simulink model "Ideal_Comparison"  (R2023b)
settings: Solver=VariableStepAuto  StartTime=0.0  StopTime=11  RelTol=1e-3
InitFcn:
  | Ld = 0.000635;
  | Lq = 0.000635;
  | Rs = 0.05;
  | Lambda_m = 0.192;
  | J = 0.011;
  | P = 4;
  | B = 0.001889;
  | Kp = 0.5;
  | Ki = 55;
libraries: slpidlib x6, spsabctodq0Lib x2, SignalEditorBlockLib x1, spspowerguiLib x1
(part 1 of 2)
settings Model: Creator=Nabil  LastModifiedBy=Nabil

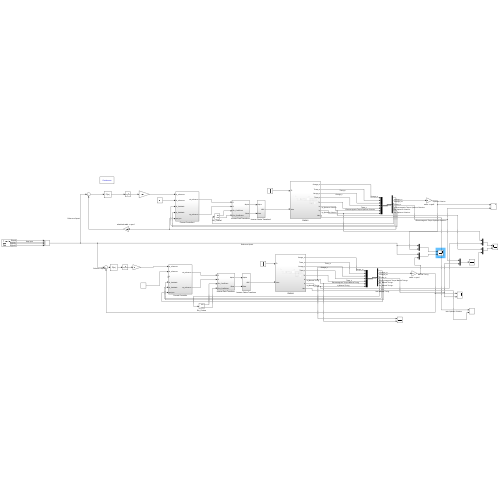
[thumbnail: Simulink's stored preview of the top-level diagram]
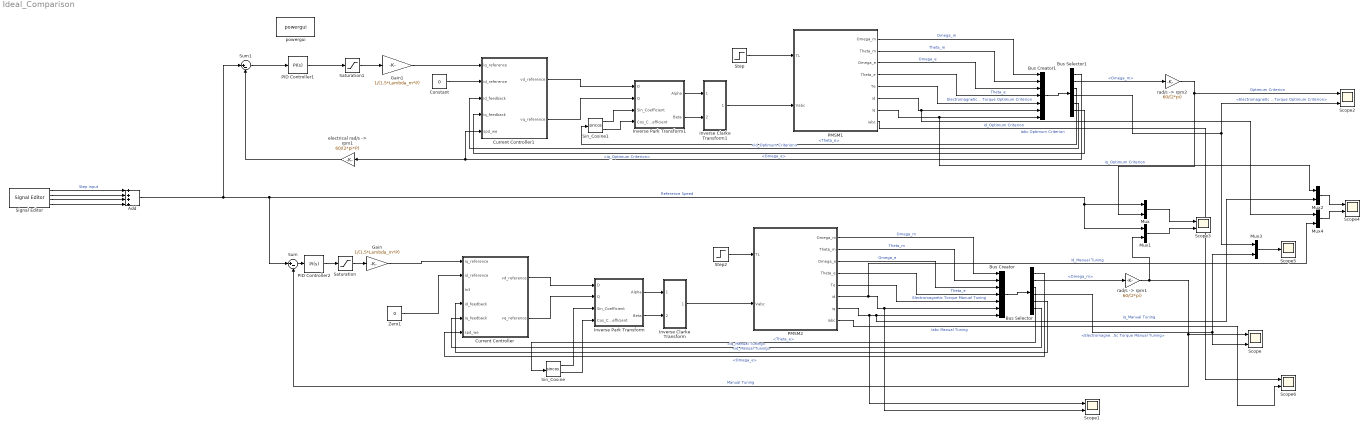
== system Ideal_Comparison ==
  Add : Sum  Inputs=++++
  Bus Creator : BusCreator  Inputs=7
  Bus Creator1 : BusCreator  Inputs=7
  Bus Selector : BusSelector  OutputSignals=Omega_e,Omega_m,Theta_e,Electromagnetic Torque Manual Tuning,id_Manual Tuning,iq_Manual Tuning
  Bus Selector1 : BusSelector  OutputSignals=Omega_e,Omega_m,Theta_e,Electromagnetic Torque Optimum Criterion,id_Optimum Criterion,iq_Optimum Criterion
  Constant : Constant  Value=0
  Current Controller : Subsystem
  Current Controller1 : Subsystem
  Gain : Gain  Gain=1/(1.5*Lambda_m*P)
  Gain1 : Gain  Gain=1/(1.5*Lambda_m*P)
  Inverse Clarke Transform : Subsystem
  Inverse Clarke Transform1 : Subsystem
  Inverse Park Transform : Subsystem
  Inverse Park Transform1 : Subsystem
  Mux{,1..4} (5 alike) : Mux  Inputs=2
  PID Controller1 : slpidlib/PID Controller  Controller=PI  Form=Parallel  TimeDomain=Continuous-time  UseExternalTs=off  SampleTime=-1  IntegratorMethod=Forward Euler  FilterMethod=Forward Euler  ControllerParametersSource=internal  P=0.218  I=2.25  UseKiTs=off  D=0  N=100  UseFilter=on  TunerSelectOption=Transfer Function Based (PID Tuner App)  InitialConditionSource=internal  InitialConditionForIntegrator=0  InitialConditionForFilter=0  DifferentiatorICPrevScaledInput=0  ExternalReset=none  TrackingMode=off  Kt=1  LimitOutput=off  SatLimitsSource=internal  UpperSaturationLimit=inf  LowerSaturationLimit=-inf  LinearizeAsGain=on  AntiWindupMode=none  Kb=1  LimitIntegrator=off  UpperIntegratorSaturationLimit=inf  LowerIntegratorSaturationLimit=-inf  POutMin=[]  POutMax=[]  IOutMin=[]  IOutMax=[]  DOutMin=[]  DOutMax=[]  NOutMin=[]  NOutMax=[]  SumOutMin=[]  SumOutMax=[]  SaturationOutMin=[]  SaturationOutMax=[]  PParamMin=[]  PParamMax=[]  IParamMin=[]  IParamMax=[]  DParamMin=[]  DParamMax=[]  NParamMin=[]  NParamMax=[]  KbParamMin=[]  KbParamMax=[]  KtParamMin=[]  KtParamMax=[]  KbOutMin=[]  KbOutMax=[]  KtOutMin=[]  KtOutMax=[]  IntegratorOutMin=[]  IntegratorOutMax=[]  FilterOutMin=[]  FilterOutMax=[]  SumI1OutMin=[]  SumI1OutMax=[]  SumI2OutMin=[]  SumI2OutMax=[]  SumI3OutMin=[]  SumI3OutMax=[]  SumI4OutMin=[]  SumI4OutMax=[]  SumDOutMin=[]  SumDOutMax=[]  DifferentiatorOutMin=[]  DifferentiatorOutMax=[]  FilterDiffOutCoefMin=[]  FilterDiffOutCoefMax=[]  ReciprocalOutMin=[]  ReciprocalOutMax=[]  SumDenOutMin=[]  SumDenOutMax=[]  SumNumOutMin=[]  SumNumOutMax=[]  DivideOutMin=[]  DivideOutMax=[]  UdiffTsProdOutMin=[]  UdiffTsProdOutMax=[]  NTsProdOutMin=[]  NTsProdOutMax=[]  UintegralTsProdOutMin=[]  UintegralTsProdOutMax=[]  UngainTsProdOutMin=[]  UngainTsProdOutMax=[]  ClampingZeroOutDataTypeStr=Inherit: Inherit via back propagation  ClampingZeroOutMin=[]  ClampingZeroOutMax=[]  FilterDenConstantOutDataTypeStr=Inherit: Inherit via back propagation  FilterDenConstantOutMin=[]  FilterDenConstantOutMax=[]  PCopyOutDataTypeStr=Inherit: Inherit via back propagation  PCopyOutMin=[]  PCopyOutMax=[]  NCopyOutDataTypeStr=Inherit: Inherit via back propagation  NCopyOutMin=[]  NCopyOutMax=[]  IntegratorContinuousStateAttributes=''  IntegratorStateMustResolveToSignalObject=off  IntegratorRTWStateStorageClass=Auto  FilterContinuousStateAttributes=''  FilterStateMustResolveToSignalObject=off  FilterRTWStateStorageClass=Auto  ParallelPVariant=InternalParameters  IdealPVariant=Disabled  IVariant=InternalParameters  DVariant=Disabled  IntegratorVariant=Continuous  SatVariant=Disabled  AWVariant=Passthrough  PCopyVariant=Disabled  TRVariant=Disabled  FdbkBlocksVariant=Forward  IdealPFdbkVariant=Disabled  SatFdbkVariant=Disabled  DerivativeFilterVariant=Disabled  NVariant=Disabled  NCopyVariant=Disabled_SignalSpec  FilterICVariant=Disabled  IntegratorICVariant=InternalICs  ExternalResetVariant=Disabled  TRSumVariant=Passthrough  SumFdbkVariant=Disabled  SumVariant=Sum_PI  TsampFilterVariant=InternalTs  TsampNgainVariant=Passthrough  TsampIntegralVariant=Disabled_SignalSpec  ExternalSaturationOutDataTypeStr=Inherit: Same as second input
  PID Controller2 : slpidlib/PID Controller  Controller=PI  Form=Parallel  TimeDomain=Continuous-time  UseExternalTs=off  SampleTime=-1  IntegratorMethod=Forward Euler  FilterMethod=Forward Euler  ControllerParametersSource=internal  P=0.3283  I=2.54  UseKiTs=off  D=0  N=100  UseFilter=on  TunerSelectOption=Transfer Function Based (PID Tuner App)  InitialConditionSource=internal  InitialConditionForIntegrator=0  InitialConditionForFilter=0  DifferentiatorICPrevScaledInput=0  ExternalReset=none  TrackingMode=off  Kt=1  LimitOutput=off  SatLimitsSource=internal  UpperSaturationLimit=inf  LowerSaturationLimit=-inf  LinearizeAsGain=on  AntiWindupMode=none  Kb=1  LimitIntegrator=off  UpperIntegratorSaturationLimit=inf  LowerIntegratorSaturationLimit=-inf  POutMin=[]  POutMax=[]  IOutMin=[]  IOutMax=[]  DOutMin=[]  DOutMax=[]  NOutMin=[]  NOutMax=[]  SumOutMin=[]  SumOutMax=[]  SaturationOutMin=[]  SaturationOutMax=[]  PParamMin=[]  PParamMax=[]  IParamMin=[]  IParamMax=[]  DParamMin=[]  DParamMax=[]  NParamMin=[]  NParamMax=[]  KbParamMin=[]  KbParamMax=[]  KtParamMin=[]  KtParamMax=[]  KbOutMin=[]  KbOutMax=[]  KtOutMin=[]  KtOutMax=[]  IntegratorOutMin=[]  IntegratorOutMax=[]  FilterOutMin=[]  FilterOutMax=[]  SumI1OutMin=[]  SumI1OutMax=[]  SumI2OutMin=[]  SumI2OutMax=[]  SumI3OutMin=[]  SumI3OutMax=[]  SumI4OutMin=[]  SumI4OutMax=[]  SumDOutMin=[]  SumDOutMax=[]  DifferentiatorOutMin=[]  DifferentiatorOutMax=[]  FilterDiffOutCoefMin=[]  FilterDiffOutCoefMax=[]  ReciprocalOutMin=[]  ReciprocalOutMax=[]  SumDenOutMin=[]  SumDenOutMax=[]  SumNumOutMin=[]  SumNumOutMax=[]  DivideOutMin=[]  DivideOutMax=[]  UdiffTsProdOutMin=[]  UdiffTsProdOutMax=[]  NTsProdOutMin=[]  NTsProdOutMax=[]  UintegralTsProdOutMin=[]  UintegralTsProdOutMax=[]  UngainTsProdOutMin=[]  UngainTsProdOutMax=[]  ClampingZeroOutDataTypeStr=Inherit: Inherit via back propagation  ClampingZeroOutMin=[]  ClampingZeroOutMax=[]  FilterDenConstantOutDataTypeStr=Inherit: Inherit via back propagation  FilterDenConstantOutMin=[]  FilterDenConstantOutMax=[]  PCopyOutDataTypeStr=Inherit: Inherit via back propagation  PCopyOutMin=[]  PCopyOutMax=[]  NCopyOutDataTypeStr=Inherit: Inherit via back propagation  NCopyOutMin=[]  NCopyOutMax=[]  IntegratorContinuousStateAttributes=''  IntegratorStateMustResolveToSignalObject=off  IntegratorRTWStateStorageClass=Auto  FilterContinuousStateAttributes=''  FilterStateMustResolveToSignalObject=off  FilterRTWStateStorageClass=Auto  ParallelPVariant=InternalParameters  IdealPVariant=Disabled  IVariant=InternalParameters  DVariant=Disabled  IntegratorVariant=Continuous  SatVariant=Disabled  AWVariant=Passthrough  PCopyVariant=Disabled  TRVariant=Disabled  FdbkBlocksVariant=Forward  IdealPFdbkVariant=Disabled  SatFdbkVariant=Disabled  DerivativeFilterVariant=Disabled  NVariant=Disabled  NCopyVariant=Disabled_SignalSpec  FilterICVariant=Disabled  IntegratorICVariant=InternalICs  ExternalResetVariant=Disabled  TRSumVariant=Passthrough  SumFdbkVariant=Disabled  SumVariant=Sum_PI  TsampFilterVariant=InternalTs  TsampNgainVariant=Passthrough  TsampIntegralVariant=Disabled_SignalSpec  ExternalSaturationOutDataTypeStr=Inherit: Same as second input
  PMSM1 : Subsystem
  PMSM2 : Subsystem
  Saturation : Saturate  UpperLimit=111  LowerLimit=-126
  Saturation1 : Saturate  UpperLimit=111  LowerLimit=-126
  Scope{,1..4,6} (6 alike) : Scope  NumInputPorts=2
  Scope5 : Scope
  Signal Editor : SignalEditorBlockLib/Signal Editor  FileName=D:\Semester 8\Files\Modeling 24_2_2024\Signal3.mat  ActiveScenario=Scenario  ActiveSignal=Signal  IsBus=off  OutputBusObjectStr=Bus: BusObject  SampleTime=0  Interpolate=off  ZeroCross=off  OutputAfterFinalValue=Setting to zero  Unit=inherit  PreserveSignalName=on  ApplySigPropsToAllScenarios=on  ApplySigPropsToAllSignals=off
  Sin_Cosine : Trigonometry  Operator=sincos
  Sin_Cosine1 : Trigonometry  Operator=sincos
  Step : Step  Before=10  After=35  SampleTime=0
  Step2 : Step  Before=10  After=35  SampleTime=0
  Sum : Sum  Inputs=|+-
  Sum1 : Sum  Inputs=|+-
  Zero1 : Constant  Value=0  OutDataTypeStr=Inherit: Inherit via back propagation
  "electrical rad/s -> rpm1" : Gain  Gain=60/(2*pi*P)
  powergui : spspowerguiLib/powergui  Priority=1  SimulationMode=Continuous  SampleTime=50e-6  frequency=60  Iterations=50  frequencyindice=0  Pbase=100e6  ErrMax=1e-4  UnitsV=kV  UnitsW=MW  buscounter=0  FunctionMessages=off  echomessages=off  EnableUseOfTLC=off  CurrentSourceSwitches=off  DisableSnubberDevices=off  DisableRonSwitches=off  DisableVfSwitches=off  DisplayEquations=off  AutomaticDiscreteSolvers=off  SolverType=Tustin/Backward Euler (TBE)  Interpol=off  ExternalGateDelay=off  methode=off  Ts=100  x0status=blocks  SPID=on  SwTol=0  HookPort=off  NonlinearTolerance=1e-4  nMaxIteration=100  ContinueOnMaxIteration=off  RestoreLinks=warning  ResistiveCurrentMeasurement=off  Frange=[0:2:500]  Ylog=off  Xlog=on  ShowGrid=off  save=off  variable=ZData  structure=0  ZoomFFT=off  StartTime=0.0  cycles=1  DisplayStyle=1  fundamental=60  FreqAxis=off  MaxFrequency=1000  frequencyindicesteady=1  RmsSteady=1  display=off
  "rad/s -> rpm1" : Gain  Gain=60/(2*pi)
  "rad/s -> rpm2" : Gain  Gain=60/(2*pi)
  wires:
  PMSM2/2(Theta_m) -> Bus Creator/2  "Theta_m"
  Bus Selector/4 -> Mux3/2, Scope/2  "<Electromagnetic Torque Manual Tuning>"
  Bus Selector/1 -> Current Controller/6(spd_we)  "<Omega_e>"
  PMSM2/3(Omega_e) -> Bus Creator/3  "Omega_e"
  PMSM2/6(id) -> Mux4/2, Scope1/2, Bus Creator/6  "id_Manual Tuning"
  PMSM2/7(iq) -> Scope1/1, Mux2/2, Bus Creator/7  "iq_Manual Tuning"
  PMSM2/5(Te) -> Bus Creator/5  "Electromagnetic Torque Manual Tuning"
  Gain/1 -> Current Controller/1(iq_reference)
  Sin_Cosine/1 -> Inverse Park Transform/3(Sin_Coefficient)
  Bus Selector/3 -> Sin_Cosine/1  "<Theta_e>"
  Inverse Park Transform/1(Alpha) -> Inverse Clarke Transform/1(Alpha)
  Current Controller/2(vq_reference) -> Inverse Park Transform/2(Q)
  Bus Selector/6 -> Current Controller/5(iq_feedback)  "<iq_Manual Tuning>"
  Bus Creator/1 -> Bus Selector/1
  Step2/1 -> PMSM2/1(TL)
  "rad/s -> rpm1"/1 -> Mux1/2, Scope/1, Sum/2  "Manual Tuning"
  Inverse Clarke Transform/1(ABC) -> PMSM2/2(Vabc)
  Sin_Cosine/2 -> Inverse Park Transform/4(Cos_Coefficient)
  Inverse Park Transform/2(Beta) -> Inverse Clarke Transform/2(Beta)
  Bus Selector/5 -> Current Controller/4(id_feedback)  "<id_Manual Tuning>"
  Bus Selector/2 -> "rad/s -> rpm1"/1  "<Omega_m>"
  PMSM2/4(Theta_e) -> Bus Creator/4  "Theta_e"
  Zero1/1 -> Current Controller/2(id_reference)
  Current Controller/1(vd_reference) -> Inverse Park Transform/1(D)
  PMSM2/1(Omega_m) -> Bus Creator/1  "Omega_m"
  PID Controller2/1 -> Saturation/1
  Sum/1 -> PID Controller2/1
  Saturation/1 -> Gain/1
  Signal Editor/1 -> Add/1  "Step input"
  PMSM1/2(Theta_m) -> Bus Creator1/2  "Theta_m"
  Bus Selector1/4 -> Mux3/1, Scope2/2  "<Electromagnetic Torque Optimum Criterion>"
  Bus Selector1/1 -> Current Controller1/5(spd_we), "electrical rad/s -> rpm1"/1  "<Omega_e>"
  PMSM1/3(Omega_e) -> Bus Creator1/3  "Omega_e"
  "electrical rad/s -> rpm1"/1 -> Sum1/2
  PMSM1/6(id) -> Mux4/1, Bus Creator1/6  "id_Optimum Criterion"
  Saturation1/1 -> Gain1/1
  Sin_Cosine1/1 -> Inverse Park Transform1/3(Sin_Coefficient)
  PMSM1/7(iq) -> Mux2/1, Bus Creator1/7  "iq_Optimum Criterion"
  PMSM1/5(Te) -> Bus Creator1/5  "Electromagnetic Torque Optimum Criterion"
  Bus Selector1/3 -> Sin_Cosine1/1  "<Theta_e>"
  Inverse Park Transform1/1(Alpha) -> Inverse Clarke Transform1/1(Alpha)
  Current Controller1/2(vq_reference) -> Inverse Park Transform1/2(Q)
  Gain1/1 -> Current Controller1/1(iq_reference)
  Bus Selector1/6 -> Current Controller1/4(iq_feedback)  "<iq_Optimum Criterion>"
  Bus Creator1/1 -> Bus Selector1/1
  Step/1 -> PMSM1/1(TL)
  "rad/s -> rpm2"/1 -> Mux/2, Scope2/1  "Optimum Criterion"
  Inverse Clarke Transform1/1(ABC) -> PMSM1/2(Vabc)
  Sin_Cosine1/2 -> Inverse Park Transform1/4(Cos_Coefficient)
  Inverse Park Transform1/2(Beta) -> Inverse Clarke Transform1/2(Beta)
  Bus Selector1/5 -> Current Controller1/3(id_feedback)  "<id_Optimum Criterion>"
  Bus Selector1/2 -> "rad/s -> rpm2"/1  "<Omega_m>"
  PMSM1/4(Theta_e) -> Bus Creator1/4  "Theta_e"
  Constant/1 -> Current Controller1/2(id_reference)
  Current Controller1/1(vd_reference) -> Inverse Park Transform1/1(D)
  PMSM1/1(Omega_m) -> Bus Creator1/1  "Omega_m"
  Mux/1 -> Scope3/1
  Mux1/1 -> Scope3/2
  Mux3/1 -> Scope5/1
  Mux4/1 -> Scope4/2
  Mux2/1 -> Scope4/1
  PMSM1/8(iabc) -> Scope6/1  "Iabc Optimum Criterion"
  PMSM2/8(iabc) -> Scope6/2  "Iabc Manual Tuning"
  Sum1/1 -> PID Controller1/1
  PID Controller1/1 -> Saturation1/1
  Signal Editor/2 -> Add/2
  Add/1 -> Sum1/1, Sum/1, Mux1/1, Mux/1  "Reference Speed"
  Signal Editor/3 -> Add/3
  Signal Editor/4 -> Add/4

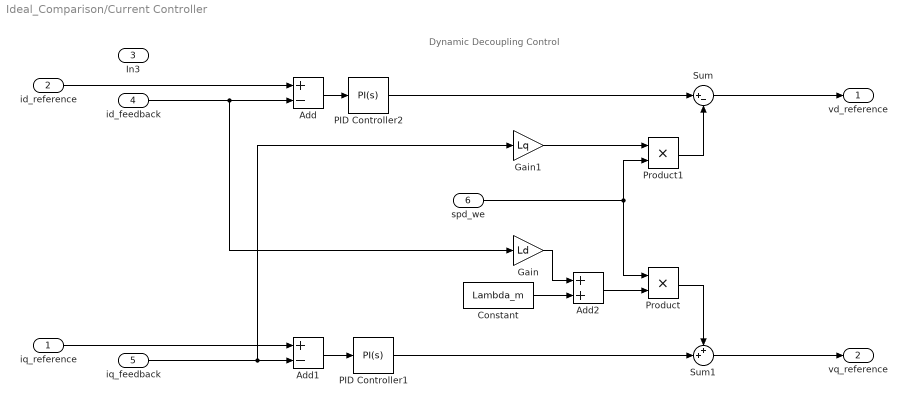
== system Ideal_Comparison/Current Controller ==
  note: Dynamic Decoupling Control
  iq_reference : Inport  SampleTime=1e-4
  id_reference : Inport  Port=2  SampleTime=1e-4
  In3 : Inport  Port=3
  id_feedback : Inport  Port=4  SampleTime=1e-4
  iq_feedback : Inport  Port=5  SampleTime=1e-4
  spd_we : Inport  Port=6  SampleTime=1e-4
  Add : Sum  Inputs=+-
  Add1 : Sum  Inputs=+-
  Add2 : Sum
  Constant : Constant  Value=Lambda_m  SampleTime=1e-4
  Gain : Gain  Gain=Ld
  Gain1 : Gain  Gain=Lq
  PID Controller1 : slpidlib/PID Controller  Controller=PI  Form=Parallel  TimeDomain=Continuous-time  UseExternalTs=off  SampleTime=-1  IntegratorMethod=Forward Euler  FilterMethod=Forward Euler  ControllerParametersSource=internal  P=0.5  I=53  UseKiTs=off  D=0  N=100  UseFilter=on  TunerSelectOption=Transfer Function Based (PID Tuner App)  InitialConditionSource=internal  InitialConditionForIntegrator=0  InitialConditionForFilter=0  DifferentiatorICPrevScaledInput=0  ExternalReset=none  TrackingMode=off  Kt=1  LimitOutput=off  SatLimitsSource=internal  UpperSaturationLimit=inf  LowerSaturationLimit=-inf  LinearizeAsGain=on  AntiWindupMode=none  Kb=1  LimitIntegrator=off  UpperIntegratorSaturationLimit=inf  LowerIntegratorSaturationLimit=-inf  POutMin=[]  POutMax=[]  IOutMin=[]  IOutMax=[]  DOutMin=[]  DOutMax=[]  NOutMin=[]  NOutMax=[]  SumOutMin=[]  SumOutMax=[]  SaturationOutMin=[]  SaturationOutMax=[]  PParamMin=[]  PParamMax=[]  IParamMin=[]  IParamMax=[]  DParamMin=[]  DParamMax=[]  NParamMin=[]  NParamMax=[]  KbParamMin=[]  KbParamMax=[]  KtParamMin=[]  KtParamMax=[]  KbOutMin=[]  KbOutMax=[]  KtOutMin=[]  KtOutMax=[]  IntegratorOutMin=[]  IntegratorOutMax=[]  FilterOutMin=[]  FilterOutMax=[]  SumI1OutMin=[]  SumI1OutMax=[]  SumI2OutMin=[]  SumI2OutMax=[]  SumI3OutMin=[]  SumI3OutMax=[]  SumI4OutMin=[]  SumI4OutMax=[]  SumDOutMin=[]  SumDOutMax=[]  DifferentiatorOutMin=[]  DifferentiatorOutMax=[]  FilterDiffOutCoefMin=[]  FilterDiffOutCoefMax=[]  ReciprocalOutMin=[]  ReciprocalOutMax=[]  SumDenOutMin=[]  SumDenOutMax=[]  SumNumOutMin=[]  SumNumOutMax=[]  DivideOutMin=[]  DivideOutMax=[]  UdiffTsProdOutMin=[]  UdiffTsProdOutMax=[]  NTsProdOutMin=[]  NTsProdOutMax=[]  UintegralTsProdOutMin=[]  UintegralTsProdOutMax=[]  UngainTsProdOutMin=[]  UngainTsProdOutMax=[]  ClampingZeroOutDataTypeStr=Inherit: Inherit via back propagation  ClampingZeroOutMin=[]  ClampingZeroOutMax=[]  FilterDenConstantOutDataTypeStr=Inherit: Inherit via back propagation  FilterDenConstantOutMin=[]  FilterDenConstantOutMax=[]  PCopyOutDataTypeStr=Inherit: Inherit via back propagation  PCopyOutMin=[]  PCopyOutMax=[]  NCopyOutDataTypeStr=Inherit: Inherit via back propagation  NCopyOutMin=[]  NCopyOutMax=[]  IntegratorContinuousStateAttributes=''  IntegratorStateMustResolveToSignalObject=off  IntegratorRTWStateStorageClass=Auto  FilterContinuousStateAttributes=''  FilterStateMustResolveToSignalObject=off  FilterRTWStateStorageClass=Auto  ParallelPVariant=InternalParameters  IdealPVariant=Disabled  IVariant=InternalParameters  DVariant=Disabled  IntegratorVariant=Continuous  SatVariant=Disabled  AWVariant=Passthrough  PCopyVariant=Disabled  TRVariant=Disabled  FdbkBlocksVariant=Forward  IdealPFdbkVariant=Disabled  SatFdbkVariant=Disabled  DerivativeFilterVariant=Disabled  NVariant=Disabled  NCopyVariant=Disabled_SignalSpec  FilterICVariant=Disabled  IntegratorICVariant=InternalICs  ExternalResetVariant=Disabled  TRSumVariant=Passthrough  SumFdbkVariant=Disabled  SumVariant=Sum_PI  TsampFilterVariant=InternalTs  TsampNgainVariant=Passthrough  TsampIntegralVariant=Disabled_SignalSpec  ExternalSaturationOutDataTypeStr=Inherit: Same as second input
  PID Controller2 : slpidlib/PID Controller  Controller=PI  Form=Parallel  TimeDomain=Continuous-time  UseExternalTs=off  SampleTime=-1  IntegratorMethod=Forward Euler  FilterMethod=Forward Euler  ControllerParametersSource=internal  P=0.5  I=53  UseKiTs=off  D=0  N=100  UseFilter=on  TunerSelectOption=Transfer Function Based (PID Tuner App)  InitialConditionSource=internal  InitialConditionForIntegrator=0  InitialConditionForFilter=0  DifferentiatorICPrevScaledInput=0  ExternalReset=none  TrackingMode=off  Kt=1  LimitOutput=off  SatLimitsSource=internal  UpperSaturationLimit=inf  LowerSaturationLimit=-inf  LinearizeAsGain=on  AntiWindupMode=none  Kb=1  LimitIntegrator=off  UpperIntegratorSaturationLimit=inf  LowerIntegratorSaturationLimit=-inf  POutMin=[]  POutMax=[]  IOutMin=[]  IOutMax=[]  DOutMin=[]  DOutMax=[]  NOutMin=[]  NOutMax=[]  SumOutMin=[]  SumOutMax=[]  SaturationOutMin=[]  SaturationOutMax=[]  PParamMin=[]  PParamMax=[]  IParamMin=[]  IParamMax=[]  DParamMin=[]  DParamMax=[]  NParamMin=[]  NParamMax=[]  KbParamMin=[]  KbParamMax=[]  KtParamMin=[]  KtParamMax=[]  KbOutMin=[]  KbOutMax=[]  KtOutMin=[]  KtOutMax=[]  IntegratorOutMin=[]  IntegratorOutMax=[]  FilterOutMin=[]  FilterOutMax=[]  SumI1OutMin=[]  SumI1OutMax=[]  SumI2OutMin=[]  SumI2OutMax=[]  SumI3OutMin=[]  SumI3OutMax=[]  SumI4OutMin=[]  SumI4OutMax=[]  SumDOutMin=[]  SumDOutMax=[]  DifferentiatorOutMin=[]  DifferentiatorOutMax=[]  FilterDiffOutCoefMin=[]  FilterDiffOutCoefMax=[]  ReciprocalOutMin=[]  ReciprocalOutMax=[]  SumDenOutMin=[]  SumDenOutMax=[]  SumNumOutMin=[]  SumNumOutMax=[]  DivideOutMin=[]  DivideOutMax=[]  UdiffTsProdOutMin=[]  UdiffTsProdOutMax=[]  NTsProdOutMin=[]  NTsProdOutMax=[]  UintegralTsProdOutMin=[]  UintegralTsProdOutMax=[]  UngainTsProdOutMin=[]  UngainTsProdOutMax=[]  ClampingZeroOutDataTypeStr=Inherit: Inherit via back propagation  ClampingZeroOutMin=[]  ClampingZeroOutMax=[]  FilterDenConstantOutDataTypeStr=Inherit: Inherit via back propagation  FilterDenConstantOutMin=[]  FilterDenConstantOutMax=[]  PCopyOutDataTypeStr=Inherit: Inherit via back propagation  PCopyOutMin=[]  PCopyOutMax=[]  NCopyOutDataTypeStr=Inherit: Inherit via back propagation  NCopyOutMin=[]  NCopyOutMax=[]  IntegratorContinuousStateAttributes=''  IntegratorStateMustResolveToSignalObject=off  IntegratorRTWStateStorageClass=Auto  FilterContinuousStateAttributes=''  FilterStateMustResolveToSignalObject=off  FilterRTWStateStorageClass=Auto  ParallelPVariant=InternalParameters  IdealPVariant=Disabled  IVariant=InternalParameters  DVariant=Disabled  IntegratorVariant=Continuous  SatVariant=Disabled  AWVariant=Passthrough  PCopyVariant=Disabled  TRVariant=Disabled  FdbkBlocksVariant=Forward  IdealPFdbkVariant=Disabled  SatFdbkVariant=Disabled  DerivativeFilterVariant=Disabled  NVariant=Disabled  NCopyVariant=Disabled_SignalSpec  FilterICVariant=Disabled  IntegratorICVariant=InternalICs  ExternalResetVariant=Disabled  TRSumVariant=Passthrough  SumFdbkVariant=Disabled  SumVariant=Sum_PI  TsampFilterVariant=InternalTs  TsampNgainVariant=Passthrough  TsampIntegralVariant=Disabled_SignalSpec  ExternalSaturationOutDataTypeStr=Inherit: Same as second input
  Product : Product
  Product1 : Product
  Sum : Sum  Inputs=|+-
  Sum1 : Sum  Inputs=++|
  vd_reference : Outport  SampleTime=1e-4  VectorParamsAs1DForOutWhenUnconnected=off
  vq_reference : Outport  Port=2  SampleTime=1e-4  VectorParamsAs1DForOutWhenUnconnected=off
  wires:
  Sum/1 -> vd_reference/1
  PID Controller2/1 -> Sum/1
  id_feedback/1 -> Gain/1, Add/2
  Add/1 -> PID Controller2/1
  iq_feedback/1 -> Gain1/1, Add1/2
  id_reference/1 -> Add/1
  Add1/1 -> PID Controller1/1
  iq_reference/1 -> Add1/1
  Sum1/1 -> vq_reference/1
  PID Controller1/1 -> Sum1/2
  Gain/1 -> Add2/1
  Constant/1 -> Add2/2
  Add2/1 -> Product/2
  spd_we/1 -> Product1/2, Product/1
  Gain1/1 -> Product1/1
  Product1/1 -> Sum/2
  Product/1 -> Sum1/1

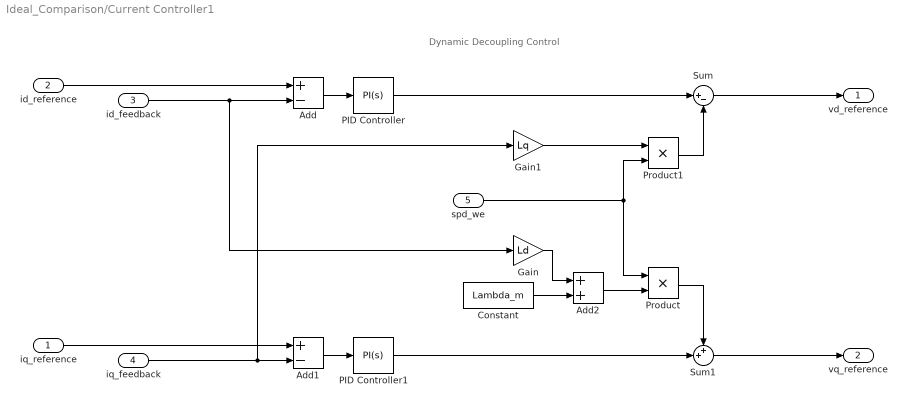
== system Ideal_Comparison/Current Controller1 ==
  note: Dynamic Decoupling Control
  iq_reference : Inport  SampleTime=1e-4
  id_reference : Inport  Port=2  SampleTime=1e-4
  id_feedback : Inport  Port=3  SampleTime=1e-4
  iq_feedback : Inport  Port=4  SampleTime=1e-4
  spd_we : Inport  Port=5  SampleTime=1e-4
  Add : Sum  Inputs=+-
  Add1 : Sum  Inputs=+-
  Add2 : Sum
  Constant : Constant  Value=Lambda_m  SampleTime=1e-4
  Gain : Gain  Gain=Ld
  Gain1 : Gain  Gain=Lq
  PID Controller : slpidlib/PID Controller  Controller=PI  Form=Parallel  TimeDomain=Continuous-time  UseExternalTs=off  SampleTime=-1  IntegratorMethod=Forward Euler  FilterMethod=Forward Euler  ControllerParametersSource=internal  P=7.9735  I=625  UseKiTs=off  D=0  N=100  UseFilter=on  TunerSelectOption=Transfer Function Based (PID Tuner App)  InitialConditionSource=internal  InitialConditionForIntegrator=0  InitialConditionForFilter=0  DifferentiatorICPrevScaledInput=0  ExternalReset=none  TrackingMode=off  Kt=1  LimitOutput=off  SatLimitsSource=internal  UpperSaturationLimit=inf  LowerSaturationLimit=-inf  LinearizeAsGain=on  AntiWindupMode=none  Kb=1  LimitIntegrator=off  UpperIntegratorSaturationLimit=inf  LowerIntegratorSaturationLimit=-inf  POutMin=[]  POutMax=[]  IOutMin=[]  IOutMax=[]  DOutMin=[]  DOutMax=[]  NOutMin=[]  NOutMax=[]  SumOutMin=[]  SumOutMax=[]  SaturationOutMin=[]  SaturationOutMax=[]  PParamMin=[]  PParamMax=[]  IParamMin=[]  IParamMax=[]  DParamMin=[]  DParamMax=[]  NParamMin=[]  NParamMax=[]  KbParamMin=[]  KbParamMax=[]  KtParamMin=[]  KtParamMax=[]  KbOutMin=[]  KbOutMax=[]  KtOutMin=[]  KtOutMax=[]  IntegratorOutMin=[]  IntegratorOutMax=[]  FilterOutMin=[]  FilterOutMax=[]  SumI1OutMin=[]  SumI1OutMax=[]  SumI2OutMin=[]  SumI2OutMax=[]  SumI3OutMin=[]  SumI3OutMax=[]  SumI4OutMin=[]  SumI4OutMax=[]  SumDOutMin=[]  SumDOutMax=[]  DifferentiatorOutMin=[]  DifferentiatorOutMax=[]  FilterDiffOutCoefMin=[]  FilterDiffOutCoefMax=[]  ReciprocalOutMin=[]  ReciprocalOutMax=[]  SumDenOutMin=[]  SumDenOutMax=[]  SumNumOutMin=[]  SumNumOutMax=[]  DivideOutMin=[]  DivideOutMax=[]  UdiffTsProdOutMin=[]  UdiffTsProdOutMax=[]  NTsProdOutMin=[]  NTsProdOutMax=[]  UintegralTsProdOutMin=[]  UintegralTsProdOutMax=[]  UngainTsProdOutMin=[]  UngainTsProdOutMax=[]  ClampingZeroOutDataTypeStr=Inherit: Inherit via back propagation  ClampingZeroOutMin=[]  ClampingZeroOutMax=[]  FilterDenConstantOutDataTypeStr=Inherit: Inherit via back propagation  FilterDenConstantOutMin=[]  FilterDenConstantOutMax=[]  PCopyOutDataTypeStr=Inherit: Inherit via back propagation  PCopyOutMin=[]  PCopyOutMax=[]  NCopyOutDataTypeStr=Inherit: Inherit via back propagation  NCopyOutMin=[]  NCopyOutMax=[]  IntegratorContinuousStateAttributes=''  IntegratorStateMustResolveToSignalObject=off  IntegratorRTWStateStorageClass=Auto  FilterContinuousStateAttributes=''  FilterStateMustResolveToSignalObject=off  FilterRTWStateStorageClass=Auto  ParallelPVariant=InternalParameters  IdealPVariant=Disabled  IVariant=InternalParameters  DVariant=Disabled  IntegratorVariant=Continuous  SatVariant=Disabled  AWVariant=Passthrough  PCopyVariant=Disabled  TRVariant=Disabled  FdbkBlocksVariant=Forward  IdealPFdbkVariant=Disabled  SatFdbkVariant=Disabled  DerivativeFilterVariant=Disabled  NVariant=Disabled  NCopyVariant=Disabled_SignalSpec  FilterICVariant=Disabled  IntegratorICVariant=InternalICs  ExternalResetVariant=Disabled  TRSumVariant=Passthrough  SumFdbkVariant=Disabled  SumVariant=Sum_PI  TsampFilterVariant=InternalTs  TsampNgainVariant=Passthrough  TsampIntegralVariant=Disabled_SignalSpec  ExternalSaturationOutDataTypeStr=Inherit: Same as second input
  PID Controller1 : slpidlib/PID Controller  Controller=PI  Form=Parallel  TimeDomain=Continuous-time  UseExternalTs=off  SampleTime=-1  IntegratorMethod=Forward Euler  FilterMethod=Forward Euler  ControllerParametersSource=internal  P=7.9735  I=625  UseKiTs=off  D=0  N=100  UseFilter=on  TunerSelectOption=Transfer Function Based (PID Tuner App)  InitialConditionSource=internal  InitialConditionForIntegrator=0  InitialConditionForFilter=0  DifferentiatorICPrevScaledInput=0  ExternalReset=none  TrackingMode=off  Kt=1  LimitOutput=off  SatLimitsSource=internal  UpperSaturationLimit=inf  LowerSaturationLimit=-inf  LinearizeAsGain=on  AntiWindupMode=none  Kb=1  LimitIntegrator=off  UpperIntegratorSaturationLimit=inf  LowerIntegratorSaturationLimit=-inf  POutMin=[]  POutMax=[]  IOutMin=[]  IOutMax=[]  DOutMin=[]  DOutMax=[]  NOutMin=[]  NOutMax=[]  SumOutMin=[]  SumOutMax=[]  SaturationOutMin=[]  SaturationOutMax=[]  PParamMin=[]  PParamMax=[]  IParamMin=[]  IParamMax=[]  DParamMin=[]  DParamMax=[]  NParamMin=[]  NParamMax=[]  KbParamMin=[]  KbParamMax=[]  KtParamMin=[]  KtParamMax=[]  KbOutMin=[]  KbOutMax=[]  KtOutMin=[]  KtOutMax=[]  IntegratorOutMin=[]  IntegratorOutMax=[]  FilterOutMin=[]  FilterOutMax=[]  SumI1OutMin=[]  SumI1OutMax=[]  SumI2OutMin=[]  SumI2OutMax=[]  SumI3OutMin=[]  SumI3OutMax=[]  SumI4OutMin=[]  SumI4OutMax=[]  SumDOutMin=[]  SumDOutMax=[]  DifferentiatorOutMin=[]  DifferentiatorOutMax=[]  FilterDiffOutCoefMin=[]  FilterDiffOutCoefMax=[]  ReciprocalOutMin=[]  ReciprocalOutMax=[]  SumDenOutMin=[]  SumDenOutMax=[]  SumNumOutMin=[]  SumNumOutMax=[]  DivideOutMin=[]  DivideOutMax=[]  UdiffTsProdOutMin=[]  UdiffTsProdOutMax=[]  NTsProdOutMin=[]  NTsProdOutMax=[]  UintegralTsProdOutMin=[]  UintegralTsProdOutMax=[]  UngainTsProdOutMin=[]  UngainTsProdOutMax=[]  ClampingZeroOutDataTypeStr=Inherit: Inherit via back propagation  ClampingZeroOutMin=[]  ClampingZeroOutMax=[]  FilterDenConstantOutDataTypeStr=Inherit: Inherit via back propagation  FilterDenConstantOutMin=[]  FilterDenConstantOutMax=[]  PCopyOutDataTypeStr=Inherit: Inherit via back propagation  PCopyOutMin=[]  PCopyOutMax=[]  NCopyOutDataTypeStr=Inherit: Inherit via back propagation  NCopyOutMin=[]  NCopyOutMax=[]  IntegratorContinuousStateAttributes=''  IntegratorStateMustResolveToSignalObject=off  IntegratorRTWStateStorageClass=Auto  FilterContinuousStateAttributes=''  FilterStateMustResolveToSignalObject=off  FilterRTWStateStorageClass=Auto  ParallelPVariant=InternalParameters  IdealPVariant=Disabled  IVariant=InternalParameters  DVariant=Disabled  IntegratorVariant=Continuous  SatVariant=Disabled  AWVariant=Passthrough  PCopyVariant=Disabled  TRVariant=Disabled  FdbkBlocksVariant=Forward  IdealPFdbkVariant=Disabled  SatFdbkVariant=Disabled  DerivativeFilterVariant=Disabled  NVariant=Disabled  NCopyVariant=Disabled_SignalSpec  FilterICVariant=Disabled  IntegratorICVariant=InternalICs  ExternalResetVariant=Disabled  TRSumVariant=Passthrough  SumFdbkVariant=Disabled  SumVariant=Sum_PI  TsampFilterVariant=InternalTs  TsampNgainVariant=Passthrough  TsampIntegralVariant=Disabled_SignalSpec  ExternalSaturationOutDataTypeStr=Inherit: Same as second input
  Product : Product
  Product1 : Product
  Sum : Sum  Inputs=|+-
  Sum1 : Sum  Inputs=++|
  vd_reference : Outport  SampleTime=1e-4  VectorParamsAs1DForOutWhenUnconnected=off
  vq_reference : Outport  Port=2  SampleTime=1e-4  VectorParamsAs1DForOutWhenUnconnected=off
  wires:
  Sum/1 -> vd_reference/1
  PID Controller/1 -> Sum/1
  id_feedback/1 -> Gain/1, Add/2
  Add/1 -> PID Controller/1
  iq_feedback/1 -> Gain1/1, Add1/2
  id_reference/1 -> Add/1
  Add1/1 -> PID Controller1/1
  iq_reference/1 -> Add1/1
  Sum1/1 -> vq_reference/1
  PID Controller1/1 -> Sum1/2
  Gain/1 -> Add2/1
  Constant/1 -> Add2/2
  Add2/1 -> Product/2
  spd_we/1 -> Product1/2, Product/1
  Gain1/1 -> Product1/1
  Product1/1 -> Sum/2
  Product/1 -> Sum1/1

== system Ideal_Comparison/Inverse Clarke Transform ==
  note: Inverse Clarke Transform
  note: Converts direct axis (alpha) component and the quadrature axis (beta) component to balanced three-phase quantities
      | The alpha and beta components are dependent on time and speed.
  Alpha : Inport
  Beta : Inport  Port=2
  Add : Sum  Inputs=-+  OutDataTypeStr=Inherit: Same as first input
  Add1 : Sum  Inputs=--  OutDataTypeStr=Inherit: Same as first input
  Gain : Gain  Gain=1/2
  Gain1 : Gain  Gain=sqrt(3)/2
  Mux : Mux  Inputs=3
  ABC : Outport  VectorParamsAs1DForOutWhenUnconnected=off
  wires:
  Beta/1 -> Gain1/1
  Mux/1 -> ABC/1
  Alpha/1 -> Mux/1, Gain/1
  Add1/1 -> Mux/3
  Gain1/1 -> Add1/2, Add/2
  Gain/1 -> Add1/1, Add/1
  Add/1 -> Mux/2

== system Ideal_Comparison/Inverse Clarke Transform1 ==
  note: Inverse Clarke Transform
  note: Converts direct axis (alpha) component and the quadrature axis (beta) component to balanced three-phase quantities
      | The alpha and beta components are dependent on time and speed.
  Alpha : Inport
  Beta : Inport  Port=2
  Add : Sum  Inputs=-+  OutDataTypeStr=Inherit: Same as first input
  Add1 : Sum  Inputs=--  OutDataTypeStr=Inherit: Same as first input
  Gain : Gain  Gain=1/2
  Gain1 : Gain  Gain=sqrt(3)/2
  Mux : Mux  Inputs=3
  ABC : Outport  VectorParamsAs1DForOutWhenUnconnected=off
  wires:
  Beta/1 -> Gain1/1
  Mux/1 -> ABC/1
  Alpha/1 -> Mux/1, Gain/1
  Add1/1 -> Mux/3
  Gain1/1 -> Add1/2, Add/2
  Gain/1 -> Add1/1, Add/1
  Add/1 -> Mux/2

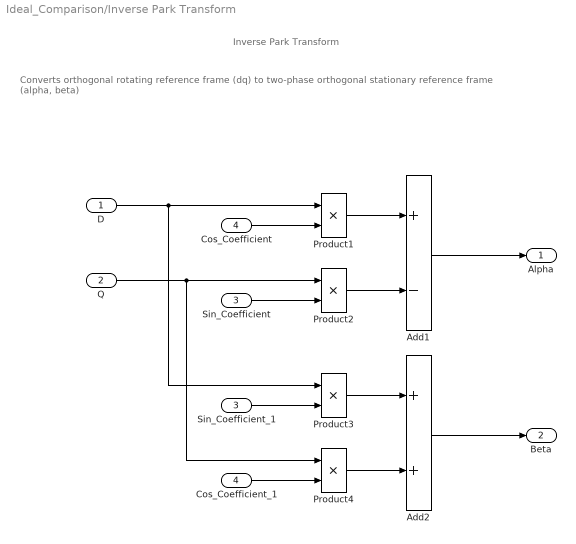
== system Ideal_Comparison/Inverse Park Transform ==
  note: Converts orthogonal rotating reference frame (dq) to two-phase orthogonal stationary reference frame (alpha, beta)
  note: Inverse Park Transform
  D : Inport
  Q : Inport  Port=2
  Sin_Coefficient : Inport  Port=3
  Cos_Coefficient : Inport  Port=4
  Add1 : Sum  Inputs=+-  OutDataTypeStr=Inherit: Same as first input
  Add2 : Sum  OutDataTypeStr=Inherit: Same as first input
  Cos_Coefficient_1 : InportShadow  Port=4
  Product{1..4} (4 alike) : Product  RndMeth=Simplest
  Sin_Coefficient_1 : InportShadow  Port=3
  Alpha : Outport  VectorParamsAs1DForOutWhenUnconnected=off
  Beta : Outport  Port=2  VectorParamsAs1DForOutWhenUnconnected=off
  wires:
  Sin_Coefficient_1/1 -> Product3/2
  Product2/1 -> Add1/2
  Cos_Coefficient_1/1 -> Product4/2
  Add2/1 -> Beta/1
  Product3/1 -> Add2/1
  Add1/1 -> Alpha/1
  Product1/1 -> Add1/1
  Product4/1 -> Add2/2
  Sin_Coefficient/1 -> Product2/2
  D/1 -> Product3/1, Product1/1
  Q/1 -> Product2/1, Product4/1
  Cos_Coefficient/1 -> Product1/2

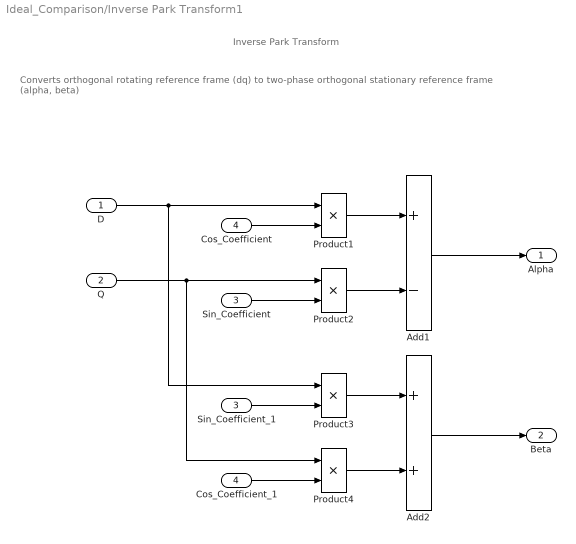
== system Ideal_Comparison/Inverse Park Transform1 ==
  note: Converts orthogonal rotating reference frame (dq) to two-phase orthogonal stationary reference frame (alpha, beta)
  note: Inverse Park Transform
  D : Inport
  Q : Inport  Port=2
  Sin_Coefficient : Inport  Port=3
  Cos_Coefficient : Inport  Port=4
  Add1 : Sum  Inputs=+-  OutDataTypeStr=Inherit: Same as first input
  Add2 : Sum  OutDataTypeStr=Inherit: Same as first input
  Cos_Coefficient_1 : InportShadow  Port=4
  Product{1..4} (4 alike) : Product  RndMeth=Simplest
  Sin_Coefficient_1 : InportShadow  Port=3
  Alpha : Outport  VectorParamsAs1DForOutWhenUnconnected=off
  Beta : Outport  Port=2  VectorParamsAs1DForOutWhenUnconnected=off
  wires:
  Sin_Coefficient_1/1 -> Product3/2
  Product2/1 -> Add1/2
  Cos_Coefficient_1/1 -> Product4/2
  Add2/1 -> Beta/1
  Product3/1 -> Add2/1
  Add1/1 -> Alpha/1
  Product1/1 -> Add1/1
  Product4/1 -> Add2/2
  Sin_Coefficient/1 -> Product2/2
  D/1 -> Product3/1, Product1/1
  Q/1 -> Product2/1, Product4/1
  Cos_Coefficient/1 -> Product1/2

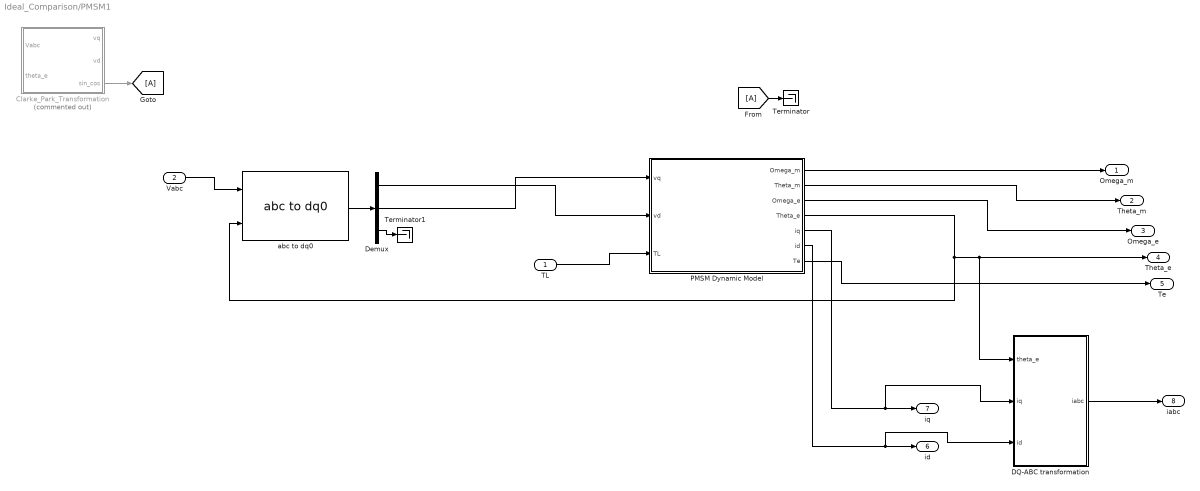
== system Ideal_Comparison/PMSM1 ==
  TL : Inport
  Vabc : Inport  Port=2
  Clarke_Park_Transformation : Subsystem  Commented=on
  DQ-ABC transformation : Subsystem
  Demux : Demux  Outputs=3
  From : From
  Goto : Goto
  PMSM Dynamic Model : Subsystem
  Terminator : Terminator
  Terminator1 : Terminator
  abc to dq0 : spsabctodq0Lib/abc to dq0  Alignment=Aligned with phase A axis
  Omega_m : Outport
  Theta_m : Outport  Port=2
  Omega_e : Outport  Port=3
  Theta_e : Outport  Port=4
  Te : Outport  Port=5
  id : Outport  Port=6
  iq : Outport  Port=7
  iabc : Outport  Port=8
  wires:
  From/1 -> Terminator/1
  PMSM Dynamic Model/2(Theta_m) -> Theta_m/1
  PMSM Dynamic Model/7(Te) -> Te/1
  PMSM Dynamic Model/6(id) -> DQ-ABC transformation/3(id), id/1
  PMSM Dynamic Model/5(iq) -> DQ-ABC transformation/2(iq), iq/1
  Clarke_Park_Transformation/3(sin_cos) -> Goto/1
  PMSM Dynamic Model/4(Theta_e) -> abc to dq0/2, DQ-ABC transformation/1(theta_e), Theta_e/1
  TL/1 -> PMSM Dynamic Model/3(TL)
  PMSM Dynamic Model/1(Omega_m) -> Omega_m/1
  PMSM Dynamic Model/3(Omega_e) -> Omega_e/1
  Vabc/1 -> abc to dq0/1
  Demux/1 -> PMSM Dynamic Model/2(vd)
  DQ-ABC transformation/1(iabc) -> iabc/1
  abc to dq0/1 -> Demux/1
  Demux/2 -> PMSM Dynamic Model/1(vq)
  Demux/3 -> Terminator1/1

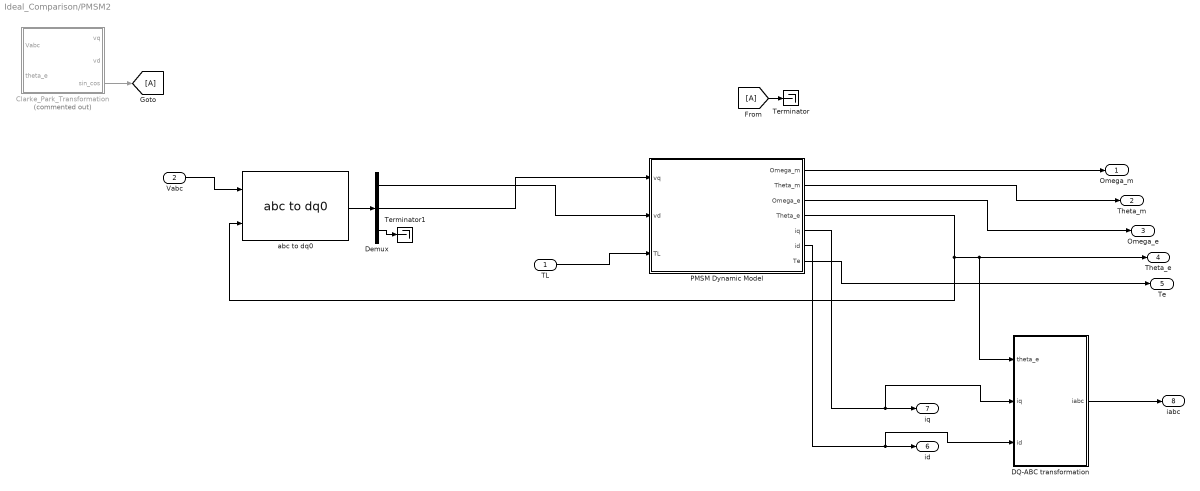
== system Ideal_Comparison/PMSM2 ==
  TL : Inport
  Vabc : Inport  Port=2
  Clarke_Park_Transformation : Subsystem  Commented=on
  DQ-ABC transformation : Subsystem
  Demux : Demux  Outputs=3
  From : From
  Goto : Goto
  PMSM Dynamic Model : Subsystem
  Terminator : Terminator
  Terminator1 : Terminator
  abc to dq0 : spsabctodq0Lib/abc to dq0  Alignment=Aligned with phase A axis
  Omega_m : Outport
  Theta_m : Outport  Port=2
  Omega_e : Outport  Port=3
  Theta_e : Outport  Port=4
  Te : Outport  Port=5
  id : Outport  Port=6
  iq : Outport  Port=7
  iabc : Outport  Port=8
  wires:
  From/1 -> Terminator/1
  PMSM Dynamic Model/2(Theta_m) -> Theta_m/1
  PMSM Dynamic Model/7(Te) -> Te/1
  PMSM Dynamic Model/6(id) -> DQ-ABC transformation/3(id), id/1
  PMSM Dynamic Model/5(iq) -> DQ-ABC transformation/2(iq), iq/1
  Clarke_Park_Transformation/3(sin_cos) -> Goto/1
  PMSM Dynamic Model/4(Theta_e) -> abc to dq0/2, DQ-ABC transformation/1(theta_e), Theta_e/1
  TL/1 -> PMSM Dynamic Model/3(TL)
  PMSM Dynamic Model/1(Omega_m) -> Omega_m/1
  PMSM Dynamic Model/3(Omega_e) -> Omega_e/1
  Vabc/1 -> abc to dq0/1
  Demux/1 -> PMSM Dynamic Model/2(vd)
  DQ-ABC transformation/1(iabc) -> iabc/1
  abc to dq0/1 -> Demux/1
  Demux/2 -> PMSM Dynamic Model/1(vq)
  Demux/3 -> Terminator1/1

== system Ideal_Comparison/PMSM1/Clarke_Park_Transformation ==
  Vabc : Inport
  theta_e : Inport  Port=2
  Clarke Transformation : Subsystem
  Constant4 : Constant  Value=0
  Mux : Mux  Inputs=2
  Park Transformation : Subsystem
  Subsystem : Subsystem
  Terminator : Terminator
  vq : Outport
  vd : Outport  Port=2
  sin_cos : Outport  Port=3
  wires:
  Vabc/1 -> Clarke Transformation/1(abc)
  Mux/1 -> sin_cos/1
  Constant4/1 -> Clarke Transformation/2(theta_degree)
  Park Transformation/2(ds_r) -> vd/1
  Clarke Transformation/3(vo_s) -> Terminator/1
  Subsystem/1(cos) -> Park Transformation/3(cos theta_e), Mux/1
  Clarke Transformation/1(vq_s) -> Park Transformation/1(qs_s)
  Clarke Transformation/2(vd_s) -> Park Transformation/2(ds_s)
  Park Transformation/1(qs_r) -> vq/1
  Subsystem/2(sin) -> Park Transformation/4(Sin theta_e), Mux/2
  theta_e/1 -> Subsystem/1(theta_e)

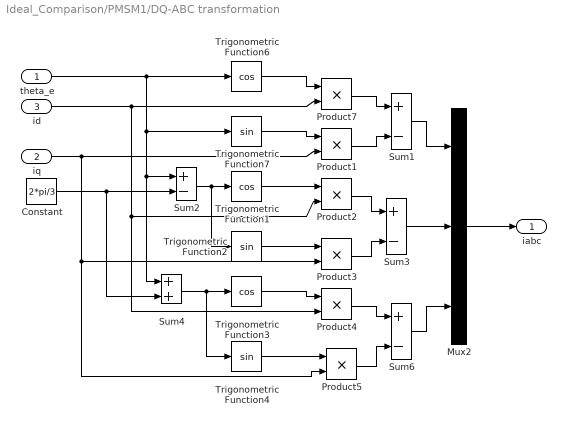
== system Ideal_Comparison/PMSM1/DQ-ABC transformation ==
  theta_e : Inport
  iq : Inport  Port=2
  id : Inport  Port=3
  Constant : Constant  Value=2*pi/3
  Mux2 : Mux  Inputs=3
  Product{1..5,7} (6 alike) : Product  InputSameDT=on  RndMeth=Zero  SaturateOnIntegerOverflow=on  OutDataTypeStr=Inherit: Same as first input
  Sum{1..3,6} (4 alike) : Sum  Inputs=+-  InputSameDT=on  SaturateOnIntegerOverflow=on  OutDataTypeStr=Inherit: Same as first input
  Sum4 : Sum  InputSameDT=on  SaturateOnIntegerOverflow=on  OutDataTypeStr=Inherit: Same as first input
  Trigonometric Function1 : Trigonometry  Operator=cos
  Trigonometric Function2 : Trigonometry
  Trigonometric Function3 : Trigonometry  Operator=cos
  Trigonometric Function4 : Trigonometry
  Trigonometric Function6 : Trigonometry  Operator=cos
  Trigonometric Function7 : Trigonometry
  iabc : Outport
  wires:
  Product2/1 -> Sum3/1
  Sum2/1 -> Trigonometric Function1/1, Trigonometric Function2/1
  iq/1 -> Product1/2, Product3/2, Product5/2
  Trigonometric Function4/1 -> Product5/1
  Constant/1 -> Sum2/2, Sum4/2
  Trigonometric Function7/1 -> Product1/1
  Mux2/1 -> iabc/1
  Sum1/1 -> Mux2/1
  Product5/1 -> Sum6/2
  Product3/1 -> Sum3/2
  Trigonometric Function3/1 -> Product4/1
  Sum4/1 -> Trigonometric Function3/1, Trigonometric Function4/1
  Trigonometric Function2/1 -> Product3/1
  Trigonometric Function6/1 -> Product7/1
  theta_e/1 -> Trigonometric Function6/1, Trigonometric Function7/1, Sum2/1, Sum4/1
  id/1 -> Product7/2, Product2/2, Product4/2
  Trigonometric Function1/1 -> Product2/1
  Sum6/1 -> Mux2/3
  Sum3/1 -> Mux2/2
  Product4/1 -> Sum6/1
  Product1/1 -> Sum1/2
  Product7/1 -> Sum1/1

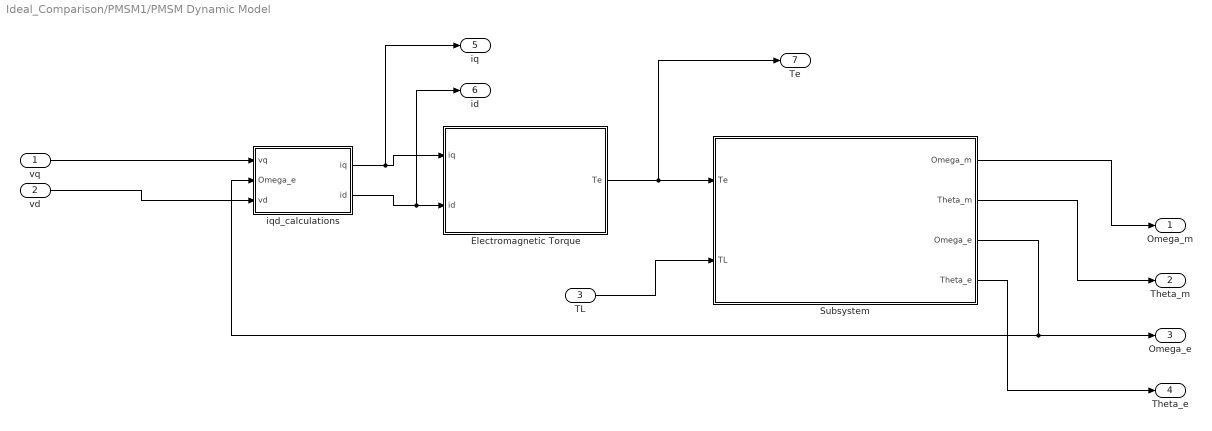
== system Ideal_Comparison/PMSM1/PMSM Dynamic Model ==
  vq : Inport
  vd : Inport  Port=2
  TL : Inport  Port=3
  Electromagnetic Torque : Subsystem
  Subsystem : Subsystem
  iqd_calculations : Subsystem
  Omega_m : Outport
  Theta_m : Outport  Port=2
  Omega_e : Outport  Port=3
  Theta_e : Outport  Port=4
  iq : Outport  Port=5
  id : Outport  Port=6
  Te : Outport  Port=7
  wires:
  Subsystem/3(Omega_e) -> Omega_e/1, iqd_calculations/2(Omega_e)
  Electromagnetic Torque/1(Te) -> Te/1, Subsystem/1(Te)
  TL/1 -> Subsystem/2(TL)
  Subsystem/4(Theta_e) -> Theta_e/1
  iqd_calculations/1(iq) -> iq/1, Electromagnetic Torque/1(iq)
  iqd_calculations/2(id) -> id/1, Electromagnetic Torque/2(id)
  Subsystem/1(Omega_m) -> Omega_m/1
  Subsystem/2(Theta_m) -> Theta_m/1
  vq/1 -> iqd_calculations/1(vq)
  vd/1 -> iqd_calculations/3(vd)

== system Ideal_Comparison/PMSM2/Clarke_Park_Transformation ==
  Vabc : Inport
  theta_e : Inport  Port=2
  Clarke Transformation : Subsystem
  Constant4 : Constant  Value=0
  Mux : Mux  Inputs=2
  Park Transformation : Subsystem
  Subsystem : Subsystem
  Terminator : Terminator
  vq : Outport
  vd : Outport  Port=2
  sin_cos : Outport  Port=3
  wires:
  Vabc/1 -> Clarke Transformation/1(abc)
  Mux/1 -> sin_cos/1
  Constant4/1 -> Clarke Transformation/2(theta_degree)
  Park Transformation/2(ds_r) -> vd/1
  Clarke Transformation/3(vo_s) -> Terminator/1
  Subsystem/1(cos) -> Park Transformation/3(cos theta_e), Mux/1
  Clarke Transformation/1(vq_s) -> Park Transformation/1(qs_s)
  Clarke Transformation/2(vd_s) -> Park Transformation/2(ds_s)
  Park Transformation/1(qs_r) -> vq/1
  Subsystem/2(sin) -> Park Transformation/4(Sin theta_e), Mux/2
  theta_e/1 -> Subsystem/1(theta_e)

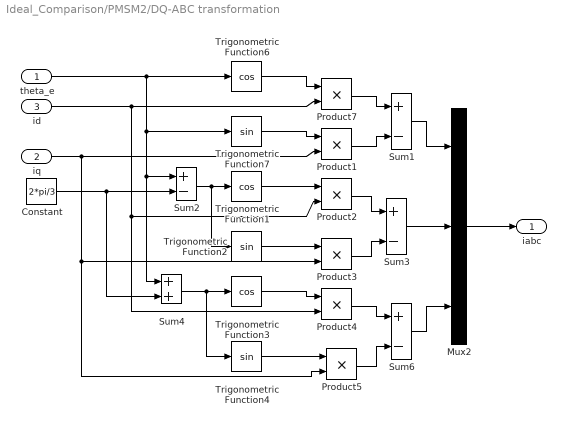
== system Ideal_Comparison/PMSM2/DQ-ABC transformation ==
  theta_e : Inport
  iq : Inport  Port=2
  id : Inport  Port=3
  Constant : Constant  Value=2*pi/3
  Mux2 : Mux  Inputs=3
  Product{1..5,7} (6 alike) : Product  InputSameDT=on  RndMeth=Zero  SaturateOnIntegerOverflow=on  OutDataTypeStr=Inherit: Same as first input
  Sum{1..3,6} (4 alike) : Sum  Inputs=+-  InputSameDT=on  SaturateOnIntegerOverflow=on  OutDataTypeStr=Inherit: Same as first input
  Sum4 : Sum  InputSameDT=on  SaturateOnIntegerOverflow=on  OutDataTypeStr=Inherit: Same as first input
  Trigonometric Function1 : Trigonometry  Operator=cos
  Trigonometric Function2 : Trigonometry
  Trigonometric Function3 : Trigonometry  Operator=cos
  Trigonometric Function4 : Trigonometry
  Trigonometric Function6 : Trigonometry  Operator=cos
  Trigonometric Function7 : Trigonometry
  iabc : Outport
  wires:
  Product2/1 -> Sum3/1
  Sum2/1 -> Trigonometric Function1/1, Trigonometric Function2/1
  iq/1 -> Product1/2, Product3/2, Product5/2
  Trigonometric Function4/1 -> Product5/1
  Constant/1 -> Sum2/2, Sum4/2
  Trigonometric Function7/1 -> Product1/1
  Mux2/1 -> iabc/1
  Sum1/1 -> Mux2/1
  Product5/1 -> Sum6/2
  Product3/1 -> Sum3/2
  Trigonometric Function3/1 -> Product4/1
  Sum4/1 -> Trigonometric Function3/1, Trigonometric Function4/1
  Trigonometric Function2/1 -> Product3/1
  Trigonometric Function6/1 -> Product7/1
  theta_e/1 -> Trigonometric Function6/1, Trigonometric Function7/1, Sum2/1, Sum4/1
  id/1 -> Product7/2, Product2/2, Product4/2
  Trigonometric Function1/1 -> Product2/1
  Sum6/1 -> Mux2/3
  Sum3/1 -> Mux2/2
  Product4/1 -> Sum6/1
  Product1/1 -> Sum1/2
  Product7/1 -> Sum1/1

== system Ideal_Comparison/PMSM2/PMSM Dynamic Model ==
  vq : Inport
  vd : Inport  Port=2
  TL : Inport  Port=3
  Electromagnetic Torque : Subsystem
  Subsystem : Subsystem
  iqd_calculations : Subsystem
  Omega_m : Outport
  Theta_m : Outport  Port=2
  Omega_e : Outport  Port=3
  Theta_e : Outport  Port=4
  iq : Outport  Port=5
  id : Outport  Port=6
  Te : Outport  Port=7
  wires:
  Subsystem/3(Omega_e) -> Omega_e/1, iqd_calculations/2(Omega_e)
  Electromagnetic Torque/1(Te) -> Te/1, Subsystem/1(Te)
  TL/1 -> Subsystem/2(TL)
  Subsystem/4(Theta_e) -> Theta_e/1
  iqd_calculations/1(iq) -> iq/1, Electromagnetic Torque/1(iq)
  iqd_calculations/2(id) -> id/1, Electromagnetic Torque/2(id)
  Subsystem/1(Omega_m) -> Omega_m/1
  Subsystem/2(Theta_m) -> Theta_m/1
  vq/1 -> iqd_calculations/1(vq)
  vd/1 -> iqd_calculations/3(vd)

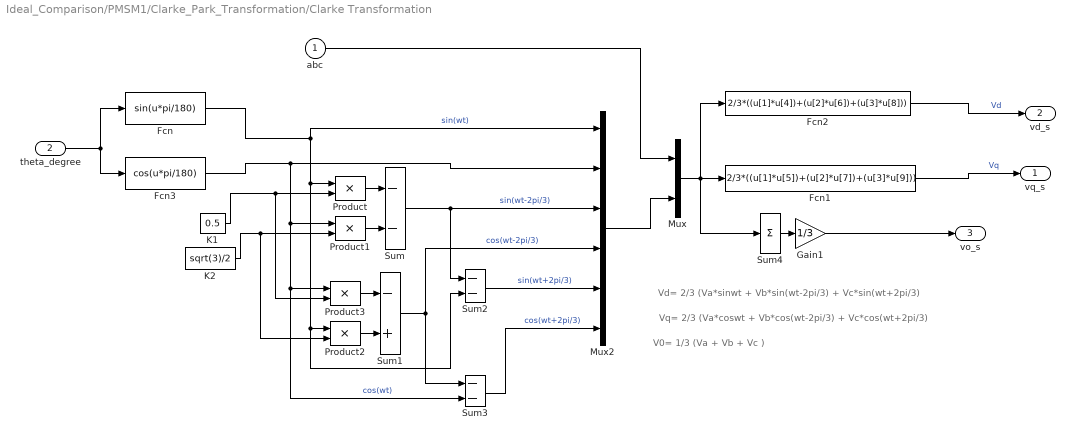
== system Ideal_Comparison/PMSM1/Clarke_Park_Transformation/Clarke Transformation ==
  note: Vd= 2/3 (Va*sinwt + Vb*sin(wt-2pi/3) + Vc*sin(wt+2pi/3)
  note: V0= 1/3 (Va + Vb + Vc )
  note: Vq= 2/3 (Va*coswt + Vb*cos(wt-2pi/3) + Vc*cos(wt+2pi/3)
  abc : Inport  PortDimensions=3
  theta_degree : Inport  Port=2
  Fcn : Fcn  Expr=sin(u*pi/180)
  Fcn1 : Fcn  Expr=2/3*((u[1]*u[5])+(u[2]*u[7])+(u[3]*u[9]))
  Fcn2 : Fcn  Expr=2/3*((u[1]*u[4])+(u[2]*u[6])+(u[3]*u[8]))
  Fcn3 : Fcn  Expr=cos(u*pi/180)
  Gain1 : Gain  Gain=1/3  SaturateOnIntegerOverflow=on  OutDataTypeStr=Inherit: Same as input  ParamDataTypeStr=Inherit: Same as input
  K1 : Constant  Value=0.5
  K2 : Constant  Value=sqrt(3)/2
  Mux : Mux  Inputs=2
  Mux2 : Mux  Inputs=6
  Product{,1..3} (4 alike) : Product  InputSameDT=on  SaturateOnIntegerOverflow=on  OutDataTypeStr=Inherit: Same as first input
  Sum : Sum  Inputs=--  InputSameDT=on  SaturateOnIntegerOverflow=on  OutDataTypeStr=Inherit: Same as first input
  Sum1 : Sum  Inputs=-+  InputSameDT=on  SaturateOnIntegerOverflow=on  OutDataTypeStr=Inherit: Same as first input
  Sum2 : Sum  Inputs=--  InputSameDT=on  SaturateOnIntegerOverflow=on  OutDataTypeStr=Inherit: Same as first input
  Sum3 : Sum  Inputs=--  InputSameDT=on  SaturateOnIntegerOverflow=on  OutDataTypeStr=Inherit: Same as first input
  Sum4 : Sum  Inputs=1  InputSameDT=on  SaturateOnIntegerOverflow=on  OutDataTypeStr=Inherit: Same as first input
  vq_s : Outport
  vd_s : Outport  Port=2
  vo_s : Outport  Port=3
  wires:
  Sum/1 -> Mux2/3, Sum2/1  "sin(wt-2pi/3)"
  Fcn1/1 -> vq_s/1  "Vq"
  Fcn3/1 -> Sum3/2, Product3/1, Product1/1, Mux2/2  "cos(wt)"
  K2/1 -> Product1/2, Product2/2
  Sum2/1 -> Mux2/5  "sin(wt+2pi/3)"
  Fcn/1 -> Product/1, Product2/1, Sum2/2, Mux2/1  "sin(wt)"
  Sum1/1 -> Mux2/4, Sum3/1  "cos(wt-2pi/3)"
  K1/1 -> Product/2, Product3/2
  Product1/1 -> Sum/2
  Product2/1 -> Sum1/2
  Mux2/1 -> Mux/2
  Product/1 -> Sum/1
  abc/1 -> Mux/1
  Sum4/1 -> Gain1/1
  Product3/1 -> Sum1/1
  Fcn2/1 -> vd_s/1  "Vd"
  Sum3/1 -> Mux2/6  "cos(wt+2pi/3)"
  theta_degree/1 -> Fcn3/1, Fcn/1
  Mux/1 -> Fcn2/1, Fcn1/1, Sum4/1
  Gain1/1 -> vo_s/1

== system Ideal_Comparison/PMSM1/Clarke_Park_Transformation/Park Transformation ==
  qs_s : Inport
  ds_s : Inport  Port=2
  cos theta_e : Inport  Port=3
  Sin theta_e : Inport  Port=4
  Add : Sum  Inputs=+-
  Add1 : Sum
  Product{,1..3} (4 alike) : Product  RndMeth=Zero
  qs_r : Outport
  ds_r : Outport  Port=2
  wires:
  cos theta_e/1 -> Product/2, Product2/2
  Sin theta_e/1 -> Product1/2, Product3/2
  Product1/1 -> Add/2
  ds_s/1 -> Product1/1, Product2/1
  Add1/1 -> ds_r/1
  Product/1 -> Add/1
  qs_s/1 -> Product/1, Product3/1
  Add/1 -> qs_r/1
  Product3/1 -> Add1/1
  Product2/1 -> Add1/2

== system Ideal_Comparison/PMSM1/Clarke_Park_Transformation/Subsystem ==
  theta_e : Inport
  Fcn : Fcn  Expr=sin(u)
  Fcn1 : Fcn  Expr=cos(u)
  cos : Outport
  sin : Outport  Port=2
  wires:
  theta_e/1 -> Fcn/1, Fcn1/1
  Fcn1/1 -> cos/1
  Fcn/1 -> sin/1

== system Ideal_Comparison/PMSM1/PMSM Dynamic Model/Electromagnetic Torque ==
  iq : Inport
  id : Inport  Port=2
  Add : Sum
  Gain : Gain  Gain=Ld-Lq
  Gain1 : Gain  Gain=(3/2)*P
  Gain2 : Gain  Gain=Lambda_m
  Product : Product
  Te : Outport
  wires:
  Add/1 -> Gain1/1
  Gain2/1 -> Add/2
  Product/1 -> Gain/1
  iq/1 -> Gain2/1, Product/1
  Gain/1 -> Add/1
  Gain1/1 -> Te/1
  id/1 -> Product/2

== system Ideal_Comparison/PMSM1/PMSM Dynamic Model/Subsystem ==
  Te : Inport
  TL : Inport  Port=2
  Gain : Gain  Gain=1/P
  Integrator : Integrator
  Mechanical_speed_calculations : Subsystem
  Omega_m : Outport
  Theta_m : Outport  Port=2
  Omega_e : Outport  Port=3
  Theta_e : Outport  Port=4
  wires:
  TL/1 -> Mechanical_speed_calculations/2(TL)
  Integrator/1 -> Theta_m/1
  Mechanical_speed_calculations/1(Omega_e) -> Gain/1, Omega_e/1
  Te/1 -> Mechanical_speed_calculations/1(Te)
  Mechanical_speed_calculations/2(Theta_e) -> Theta_e/1
  Gain/1 -> Integrator/1, Omega_m/1

== system Ideal_Comparison/PMSM1/PMSM Dynamic Model/iqd_calculations ==
  vq : Inport
  Omega_e : Inport  Port=2
  vd : Inport  Port=3
  id_calculations : Subsystem
  iq_calculations : Subsystem
  iq : Outport
  id : Outport  Port=2
  wires:
  vq/1 -> iq_calculations/1(vq)
  id_calculations/1(id) -> id/1, iq_calculations/3(id)
  Omega_e/1 -> iq_calculations/2(Omega_e), id_calculations/2(Omega_e)
  iq_calculations/1(iq) -> iq/1, id_calculations/3(iq)
  vd/1 -> id_calculations/1(vd)

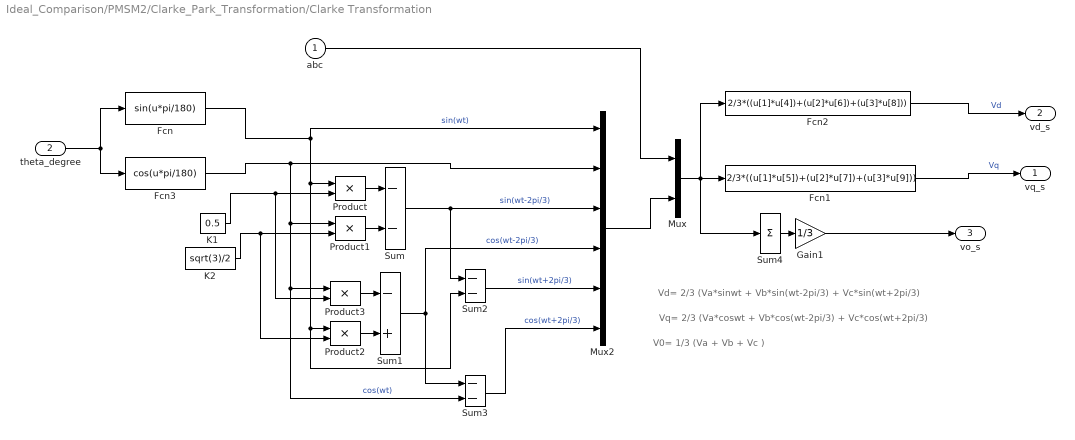
== system Ideal_Comparison/PMSM2/Clarke_Park_Transformation/Clarke Transformation ==
  note: Vd= 2/3 (Va*sinwt + Vb*sin(wt-2pi/3) + Vc*sin(wt+2pi/3)
  note: V0= 1/3 (Va + Vb + Vc )
  note: Vq= 2/3 (Va*coswt + Vb*cos(wt-2pi/3) + Vc*cos(wt+2pi/3)
  abc : Inport  PortDimensions=3
  theta_degree : Inport  Port=2
  Fcn : Fcn  Expr=sin(u*pi/180)
  Fcn1 : Fcn  Expr=2/3*((u[1]*u[5])+(u[2]*u[7])+(u[3]*u[9]))
  Fcn2 : Fcn  Expr=2/3*((u[1]*u[4])+(u[2]*u[6])+(u[3]*u[8]))
  Fcn3 : Fcn  Expr=cos(u*pi/180)
  Gain1 : Gain  Gain=1/3  SaturateOnIntegerOverflow=on  OutDataTypeStr=Inherit: Same as input  ParamDataTypeStr=Inherit: Same as input
  K1 : Constant  Value=0.5
  K2 : Constant  Value=sqrt(3)/2
  Mux : Mux  Inputs=2
  Mux2 : Mux  Inputs=6
  Product{,1..3} (4 alike) : Product  InputSameDT=on  SaturateOnIntegerOverflow=on  OutDataTypeStr=Inherit: Same as first input
  Sum : Sum  Inputs=--  InputSameDT=on  SaturateOnIntegerOverflow=on  OutDataTypeStr=Inherit: Same as first input
  Sum1 : Sum  Inputs=-+  InputSameDT=on  SaturateOnIntegerOverflow=on  OutDataTypeStr=Inherit: Same as first input
  Sum2 : Sum  Inputs=--  InputSameDT=on  SaturateOnIntegerOverflow=on  OutDataTypeStr=Inherit: Same as first input
  Sum3 : Sum  Inputs=--  InputSameDT=on  SaturateOnIntegerOverflow=on  OutDataTypeStr=Inherit: Same as first input
  Sum4 : Sum  Inputs=1  InputSameDT=on  SaturateOnIntegerOverflow=on  OutDataTypeStr=Inherit: Same as first input
  vq_s : Outport
  vd_s : Outport  Port=2
  vo_s : Outport  Port=3
  wires:
  Sum/1 -> Mux2/3, Sum2/1  "sin(wt-2pi/3)"
  Fcn1/1 -> vq_s/1  "Vq"
  Fcn3/1 -> Sum3/2, Product3/1, Product1/1, Mux2/2  "cos(wt)"
  K2/1 -> Product1/2, Product2/2
  Sum2/1 -> Mux2/5  "sin(wt+2pi/3)"
  Fcn/1 -> Product/1, Product2/1, Sum2/2, Mux2/1  "sin(wt)"
  Sum1/1 -> Mux2/4, Sum3/1  "cos(wt-2pi/3)"
  K1/1 -> Product/2, Product3/2
  Product1/1 -> Sum/2
  Product2/1 -> Sum1/2
  Mux2/1 -> Mux/2
  Product/1 -> Sum/1
  abc/1 -> Mux/1
  Sum4/1 -> Gain1/1
  Product3/1 -> Sum1/1
  Fcn2/1 -> vd_s/1  "Vd"
  Sum3/1 -> Mux2/6  "cos(wt+2pi/3)"
  theta_degree/1 -> Fcn3/1, Fcn/1
  Mux/1 -> Fcn2/1, Fcn1/1, Sum4/1
  Gain1/1 -> vo_s/1

== system Ideal_Comparison/PMSM2/Clarke_Park_Transformation/Park Transformation ==
  qs_s : Inport
  ds_s : Inport  Port=2
  cos theta_e : Inport  Port=3
  Sin theta_e : Inport  Port=4
  Add : Sum  Inputs=+-
  Add1 : Sum
  Product{,1..3} (4 alike) : Product  RndMeth=Zero
  qs_r : Outport
  ds_r : Outport  Port=2
  wires:
  cos theta_e/1 -> Product/2, Product2/2
  Sin theta_e/1 -> Product1/2, Product3/2
  Product1/1 -> Add/2
  ds_s/1 -> Product1/1, Product2/1
  Add1/1 -> ds_r/1
  Product/1 -> Add/1
  qs_s/1 -> Product/1, Product3/1
  Add/1 -> qs_r/1
  Product3/1 -> Add1/1
  Product2/1 -> Add1/2

== system Ideal_Comparison/PMSM2/Clarke_Park_Transformation/Subsystem ==
  theta_e : Inport
  Fcn : Fcn  Expr=sin(u)
  Fcn1 : Fcn  Expr=cos(u)
  cos : Outport
  sin : Outport  Port=2
  wires:
  theta_e/1 -> Fcn/1, Fcn1/1
  Fcn1/1 -> cos/1
  Fcn/1 -> sin/1

== system Ideal_Comparison/PMSM2/PMSM Dynamic Model/Electromagnetic Torque ==
  iq : Inport
  id : Inport  Port=2
  Add : Sum
  Gain : Gain  Gain=Ld-Lq
  Gain1 : Gain  Gain=(3/2)*P
  Gain2 : Gain  Gain=Lambda_m
  Product : Product
  Te : Outport
  wires:
  Add/1 -> Gain1/1
  Gain2/1 -> Add/2
  Product/1 -> Gain/1
  iq/1 -> Gain2/1, Product/1
  Gain/1 -> Add/1
  Gain1/1 -> Te/1
  id/1 -> Product/2

== system Ideal_Comparison/PMSM2/PMSM Dynamic Model/Subsystem ==
  Te : Inport
  TL : Inport  Port=2
  Gain : Gain  Gain=1/P
  Integrator : Integrator
  Mechanical_speed_calculations : Subsystem
  Omega_m : Outport
  Theta_m : Outport  Port=2
  Omega_e : Outport  Port=3
  Theta_e : Outport  Port=4
  wires:
  TL/1 -> Mechanical_speed_calculations/2(TL)
  Integrator/1 -> Theta_m/1
  Mechanical_speed_calculations/1(Omega_e) -> Gain/1, Omega_e/1
  Te/1 -> Mechanical_speed_calculations/1(Te)
  Mechanical_speed_calculations/2(Theta_e) -> Theta_e/1
  Gain/1 -> Integrator/1, Omega_m/1
